simulink model "fxpdemo_approx"  (Simulink 7.6)
settings: Solver=FixedStepDiscrete  StartTime=0.0  StopTime=1  FixedStep=0.01  RelTol=1e-3
InitFcn:
  | if ~exist('xuneven') || ~exist('yuneven') || ~exist('xeven') || ~exist('yeven') || ~exist('xpow2') || ~exist('ypow2')
  |  funcStr = 'sin(2*pi*x)';
  |  xmin = 0; xmax = 0.25;
  |  xdt    = ufix(16); xscale = 2^(-16);
  |  ydt    = sfix(16); yscale = 2^(-14);
  |  errMax  = 2^(-8);
  |  nPtsMax = 21;
  |  rndMeth = 'Floor';
  |  [xuneven,yuneven] = fixpt_look1_func_approx(funcStr,xmin,xmax,xdt,xscale,ydt,yscale,rndMeth,errMax,[]);
  |  [xeven,yeven] = fixpt_look1_func_approx(funcStr,xmin,xmax,xdt,xscale,ydt,yscale,rndMeth,errMax,[],'even');
  |  [xpow2,ypow2] = fixpt_look1_func_approx(funcStr,xmin,xmax,xdt,xscale,ydt,yscale,rndMeth,errMax,[],'pow2');
  | end
values from neighbouring files (symbols this model uses):
  xeven = [1 2]    [fxpdemo_approx_sin.m]
  xpow2 = [1 2]    [fxpdemo_approx_sin.m]
  yeven = [1 2]    [fxpdemo_approx_sin.m]
  ypow2 = [1 2]    [fxpdemo_approx_sin.m]
undefined symbols (not defined in the file or in its folder): xuneven, yuneven
libraries: simulink x1
settings Model: MinMaxOverflowLogging=MinMaxAndOverflow  Creator=The MathWorks Inc.  CovMetricSettings=d  ExtModeAutoUpdateStatusClock=off  TunableVars=xuneven,yeven,ypow2,yuneven  TunableVarsStorageClass=ExportedGlobal,ExportedGlobal,ExportedGlobal,ExportedGlobal  TunableVarsTypeQualifier=,,,
settings SolverCC: InsertRTBMode=Auto
settings DataIOCC: SaveOutput=off  SaveTime=off  SignalLoggingName=sigsOut
settings OptimizationCC: BooleanDataType=off  InlineParams=on  InlineInvariantSignals=on  InitFltsAndDblsToZero=on
settings DebuggingCC: SaveWithParameterizedLinksMsg=none  SignalResolutionControl=TryResolveAllWithWarning  SolverPrmCheckMsg=none  MultiTaskDSMMsg=warning  MultiTaskCondExecSysMsg=none  SigSpecEnsureSampleTimeMsg=none  ParameterDowncastMsg=warning  ParameterOverflowMsg=warning  ParameterPrecisionLossMsg=none  StrictBusMsg=None
settings HardwareCC: TargetUnknown=on
settings RTWCC: IncludeERTFirstTime=on
settings GRTTargetCC: TargetFcnLib=ansi_tfl_tmw.mat

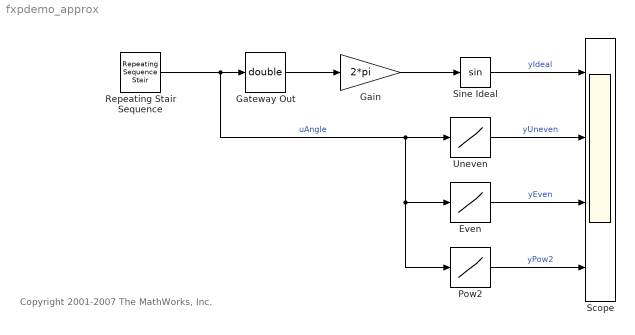
== system fxpdemo_approx ==
  note: Copyright 2001-2007 The MathWorks, Inc.
  Even : Lookup_n-D  NumberOfTableDimensions=1  BreakpointsForDimension1=xeven  IndexSearchMethod=Evenly spaced points  Table=yeven  ExtrapMethod=None - Clip  OutDataTypeStr=fixdt(1,16,14)  InputSameDT=on
      settings: AttributesFormatString=Sine Approx
  Gain : Gain  Gain=2*pi  SaturateOnIntegerOverflow=on  OutDataTypeStr=Inherit: Same as input  ParamDataTypeStr=Inherit: Same as input
  Gateway Out : DataTypeConversion  OutDataTypeStr=double
  Pow2 : Lookup_n-D  NumberOfTableDimensions=1  BreakpointsForDimension1=xpow2  IndexSearchMethod=Evenly spaced points  Table=ypow2  ExtrapMethod=None - Clip  OutDataTypeStr=fixdt(1,16,14)  InputSameDT=on
      settings: AttributesFormatString=Sine Approx
  Repeating Stair Sequence : simulink/Sources/Repeating Sequence Stair  SystemSampleTime=-1  OutValues=linspace(0,0.25,100).'  tsamp=-1  OutMin=[]  OutMax=[]  OutDataTypeStr=fixdt(0,16,14)  OutputDataTypeScalingMode=Specify via dialog  OutDataType=ufix(16)  ConRadixGroup=Use specified scaling  OutScaling=2^-14
  Scope : Scope  NumInputPorts=4
      settings: TimeRange=1  YMin=0~0~0~0  YMax=1~1~1~1
  Sine Ideal : Trigonometry
  Uneven : Lookup_n-D  NumberOfTableDimensions=1  BreakpointsForDimension1=xuneven  Table=yuneven  ExtrapMethod=None - Clip  OutDataTypeStr=fixdt(1,16,14)  InputSameDT=on
      settings: AttributesFormatString=Sine Approx
  wires:
  Repeating Stair Sequence/1 -> Even/1, Pow2/1, Uneven/1, Gateway Out/1  "uAngle"
  Gain/1 -> Sine Ideal/1
  Gateway Out/1 -> Gain/1
  Sine Ideal/1 -> Scope/1  "yIdeal"
  Uneven/1 -> Scope/2  "yUneven"
  Even/1 -> Scope/3  "yEven"
  Pow2/1 -> Scope/4  "yPow2"
